simulink model "SLUGS2"  (R2015a)
settings: Solver=FixedStepDiscrete  StartTime=0.0  StopTime=10.0  FixedStep=T  RelTol=1e-3
PreLoadFcn:
  | %T = 0.0025;
  | MavlinkBus;
  | mcuInit;
  | % Baro Altitude Computation
  | % =========================
  | %basePressure = 98192.64;
  | %baseTemp = 288.215;
  | %lapseRate = -0.00198122;
  | %baseHeight = 0;
values from neighbouring files (symbols this model uses):
  apSampleTime = 0.01    [mcuInit.m]
  latlong_WP = 1    [mcuInit.m]
  mavlink_attitude_t = Simulink.Bus    [MavlinkBusMarcello.m]
  mavlink_gps_raw_int_t = Simulink.Bus    [MavlinkBus.m]    (also in MavlinkBusMarcello.m)
  mavlink_raw_imu_t = Simulink.Bus    [MavlinkBus.m]    (also in MavlinkBusMarcello.m)
  mavlink_scaled_pressure_t = Simulink.Bus    [MavlinkBus.m]    (also in MavlinkBusMarcello.m)
  mavlink_servo_output_raw_t = Simulink.Bus    [MavlinkBusMarcello.m]
  mavlink_slugs_navigation_t = Simulink.Bus    [MavlinkBusMarcello.m]
  mavlink_sys_status_t = Simulink.Bus    [MavlinkBus.m]    (also in MavlinkBusMarcello.m)
  SYS_ID_DEF = mpt.Parameter    [mcuInit.m]
  T = 0.01    [mcuInit.m]
  Xpoints = [0 0]    [mcuInit.m]
  Ypoints = [0 0]    [mcuInit.m]
  Zpoints = [0 0]    [mcuInit.m]
undefined symbols (not defined in the file or in its folder): A0, A14, A15, A2, A3, A4, A5, A6, accBiasRateLimit, B0, bankCommandLimit, barAdjust, baroCutoff, baroCutTemp, baseHeight, baseTemp, bdt, cubeAccelGain16405, cubeGyroGain16405, cubeMagGain16405, D0, D11, D7, D8, daLimit, data, daTrimMax, daTrimMin, deLimit, deTrimMax, deTrimMin, drLimit, drTrimMax, drTrimMin, dtLimit, dtTrimMax, dtTrimMin, F2, F3, G0, G13, G15, gaind, GS_location, gyroBiasRateLimit, imuOffset_xacc, imuOffset_xgyro, imuOffset_yacc, imuOffset_ygyro, imuOffset_zacc, imuOffset_zgyro, IPStar, ISA_g, Max, maxAcc, MaxDwnPthStar, maxDynPressure, maxEta, mdt, mlParamInterface ... (+34)
undefined symbols (not defined in the file): baroOffset, baroScale, barTGain1, barTGain2, barTMean1, barTMean2, bda, bde, bdr, bICda, bICde, bICdr, bICdt, derivativesConstant, lapseRate, lowRateSensorCutoff, mainSensorCutoff, mda, mde, mdr, mICda, mICde, mICdr, mICdt, pitotOffset, pitotScale, pitTGain1, pitTGain2, pitTMean1, pitTMean2, powerOffset, powerScale, pressureSensorCutoff, tempOffset, tempScale, vzCutoff, xCutoff, yCutoff
libraries: MCHP_Blockset x151, simulink x84, SLUGS_Library x31, aerolibconvert2 x6, aerolibutil x4, aerolibtransform2 x3, dspmtrx3 x2, aerolibobsolete x2
(part 16 of 24)

== system SLUGS2/Sensor_Data_Adapter/Sensor Suite/ GPS is Ublox ==
  Produce the GPS Main Data and update the AP State (lat lon hei cog sog) [gpsUblox.c]1 : MCHP_Blockset/User Functions/C Function Call  ParseFilesChkbx=on  ListFunctions1=Custom Function  Function1=void getGpsUbloxData(real32_T* y1);  AddHeaderDeclaration=on  Function1Type=when block is updated (default)  FctReturnBlockOut=off  Fct1BlockOut=y1[5]  DataCollected="s.chksm=reshape({ '638530-ספט-2016 08:52:24','251930-ספט-2016 08:52:57','1656312-אוק-2016 11:02:56','3862408-אוק-2016 23:39:15','360330-ספט-2016 08:52:57','7293730-ספט-2016 08:52:57','954930-ספט-2016 08:52:57','296108-אוק-2016 23:39:15','278130-ספט-2016 08:52:57','556030-ספט-2016 08:52:57','963230-ספט-2016 08:52:57','1122730-ספט-2016 08:52:57','372430-ספט-2016 08:52:57','998830-ספט-2016 08:52:57','522508-אוק-2016 23:39:15'},1,15);s.File1=reshape({ '  void  newCircBuffer(CBRef cB)','  void  freeCircBuffer(CBRef* cB)','  void  freeCircBuffer(CBRef* cB)',' unsigned int  getLength(CBRef cB)','  int  readHead(CBRef cB)','  int  readTail(CBRef cB)',' unsigned char  peak(CBRef cB)',' unsigned char  readFront(CBRef cB)',' unsigned char  writeBack(CBRef cB, unsigned char data)','  void  makeEmpty(CBRef cB)','  void  printCircBuf(CBRef cB)'},1,11);s.File2=reshape({ '  void  uartBufferInit(void)','  void  __attribute__((__interrupt__, no_auto_psv)) _U4RXInterrupt(void)','  void  getGPSRawData(unsigned char* gpsBuffer)',' unsigned char  isGPSNovatel(void)'},1,4);s.File3=reshape({ '  char  hex2char(char halfhex)','  float  degMinToDeg(unsigned char degrees, float minutes)',' unsigned char  gpsUbloxSeparate(unsigned char* outStream)','  void  gpsUbloxParse(void)','  void  getGpsUbloxMainData(float* data)','  void  getGpsUbloxData(float* data)','  char  gpSmbl(char symbl)',' unsigned char  myTokenizer(char* stringToTokenize, char token, char * returnToken)','  void  parseRMC(unsigned char* stream)','  void  parseGGA(unsigned char* stream)',' unsigned char  getChecksum(unsigned char* sentence, unsigned char size)','  void  gpsDebugMsg(unsigned char buf)'},1,12);s.File4=reshape({ '  void  uartMavlinkBufferInit(void)','  void __attribute__((__interrupt__,__auto_psv__)) _U1RXInterrupt(void)','  uint8_t  isFinite(float s)','  void  InitParameterInterface(void)','  void  protDecodeMavlink(void)','  uint16_t  MissionInterfaceResponse(uint8_t system_id, uint8_t component_id)','  uint16_t  ParameterInterfaceResponse(uint8_t system_id, uint8_t component_id)','  uint16_t  PackHeartBeat(uint8_t system_id, uint8_t component_id)','  uint16_t  PackTextMsg(uint8_t system_id, uint8_t component_id, unsigned char buf)','  uint16_t  PackRawIMU(uint8_t system_id, uint8_t component_id, mavlink_raw_imu_t mlRawIMUData ,uint32_t time_usec)','  uint16_t  PackRawAttitude(uint8_t system_id, uint8_t component_id, mavlink_attitude_t mlAttitudeData ,uint32_t time_usec)','  uint16_t  PackGpsRawInt(uint8_t system_id, uint8_t component_id, mavlink_gps_raw_int_t mlRawGpsDataInt ,uint32_t time_usec)','  uint16_t  PackScaledPressure(uint8_t system_id, uint8_t component_id, mavlink_scaled_pressure_t mlAirData ,uint32_t time_usec)','  uint16_t  PackSysStatus(uint8_t system_id, uint8_t component_id, mavlink_sys_status_t mlSysStatus)','  uint16_t  PackRawServo(uint8_t system_id, uint8_t component_id, mavlink_servo_output_raw_t mlPwmCommands ,uint32_t time_usec)','  uint16_t  HIL_PackRawServo(uint8_t system_id, uint8_t component_id, mavlink_servo_output_raw_t mlPwmCommands ,uint32_t time_usec)','  uint16_t  PackRawRC(uint8_t system_id, uint8_t component_id, mavlink_rc_channels_raw_t mlRC_Commands ,uint32_t time_usec)','  uint16_t  PackVFR_HUD(uint8_t system_id, uint8_t component_id, mavlink_vfr_hud_t mlVfr_hud ,uint32_t time_usec)','  char  sendQGCDebugMessage(const char * dbgMessage, char severity, unsigned char* bytesToAdd, char positionStart)','  void  TxN_Data_OverU1(uint16_t N)','  void  TxN_Data_OverU4(uint16_t N)'},1,21);s.File5=reshape({ '  float  myAtan2(float num, float denom)','  float  myPow(float x, float toTheN)','  float  mySqrt(float x)','  float  myAbs(float x)','  float  myAtan(float x)','  float  myAsin(float x)','  float  mySin(float x)','  float  myCos(float x)','  float  myTan(float x)','  float  myAcos(float x)','  float  myExp(float x)','  void  hugeDelay(void)','  void  smallDelay(void)','  void  tinyDelay(void)','  void  printToUart2(const char *fmt, ...)'},1,15);s.File6=reshape({ '  void  sendTelemetryMavlink(unsigned char* dataOut)','  void  uart2Init(void)','  void  gsRead(unsigned char* gsChunk)','  void  prepareTelemetryMavlink(unsigned char* dataOut)','  void  prepareTelemetryMavlink(unsigned char* dataOut)','  void  sendTelemetryMavlink(unsigned char* dataOut)','  void  copyBufferToDMA1(unsigned char size)','  void  send2GS(unsigned char* protData)','  uint8_t  clearWaypointsFrom(uint8_t startingWp)','  void  addMessageToSpiOut(mavlink_message_t* msg)'},1,10);s.File7={ '  void  populateParameterInterface(void)'};s.File8={ '  void  mavlinkInit(void)'};s.File9=reshape({ '  void  updatePWM(unsigned short * PWMData)','  void  updatePWMTrim(unsigned short PWMData, unsigned char channel)','  void  updateLoad(uint8_t mcuLoad)','  void  updateEuler(float* newEuler)','  void  updatePQR(float* newPQR)',' unsigned char  getHilOnOff(void)','  uint8_t  getLightsOnOff(void)','  uint8_t  getLightsDayNight(void)','  void  updateVISensor(uint16_t* data)','  void  updatePTZ(int16_t* ptz)'},1,10);s.File10=reshape({ '  void  updateRawADCData(int16_t* adcData)','  void  updateAirData(float* airData)','  void  updateLoadData(uint8_t load, uint16_t mvPower)','  void  updateAttitude(float * attitudeData)','  void  getGSLocation(float* altLatLon)','  void  updateTimeStamp(uint32_t timeSt)','  void  updatePosition(float * posData)','  void  updatePilotConsole(uint16_t * pilData)','  void  updateDiagnosticFl(float* diagFl)','  void  updateDiagnosticSh(int16_t* diagSh)','  void  updateBias(float * biasData)','  void  updateSensorData(float* sens)','  uint8_t  isFixValid(void)','  void  updateSensorDiag(float* diag)'},1,14);s.File11=reshape({ '  void  gpsInit(void)','  void  gpsParse(uint8_t* dataStream)','  void  updateStatus(uint8_t* completeMessage)','  void  updatePositionData(uint8_t* completeMessage)','  void  updateVelocityData(uint8_t* completeMessage)','  void  updateTimeData(uint8_t* completeMessage)','  void  getGpsMainData(float* data)','  uint32_t  CRC32Value(int32_t i)','  uint32_t  CalculateBlockCRC32(uint32_t ulCount, uint8_t *ucBuffer)','  uint16_t  charsToUint16(uint8_t* data)','  uint32_t  charsToUint32(uint8_t* data)','  float  charsToFloat(uint8_t* data)','  double  charsToDouble(uint8_t* data)'},1,13);s.File12=reshape({ '  void  getMidLevelCommands(float* commands)',' unsigned char  isApManual(uint16_t failsafe)','  float  getParamIdx(unsigned char idx)','  void  getRangeOfParams(uint8_t startIdx, uint8_t endIdx, float* parameters)','  float  getDynamic(void)','  void  getAttitude(float* attitude)','  void  getXYZ(float* xyz)','  void  getVned(float* xyz)','  uint8_t  getMaxWp(void)',' unsigned char  isWpFly(void)',' unsigned char  isPassthrough(void)','  void  setDiagnosticFloat(float * flValues)','  void  setDiagnosticShort(int16_t* shValues)','  void  getWP(unsigned char idx, float* WPpos)','  void  setLogFloat1(float * flValues)','  void  setLogFloat2(float * flValues)',' unsigned char  getApControlType(void)',' unsigned char  getPassValues(uint8_t* pasVals)','  void  setCurrentCommands(float airSpeed)','  void  getCurrentGPSPos(float* latLonAlt)','  void  setNavLong(float* values)','  void  setNavLat(float* values)','  void  setNavNav(float* values)','  void  getAccels(float * accels)','  void  getAccBias(float * bias)','  void  getRTB(uint8_t* rtb)','  void  getMobileLocation(float* loc)','  uint8_t  getNavMode(void)','  void  getISRLocation(float* loc)','  uint8_t  getISRCameraOption1(void)',' unsigned short  meanFilter5(unsigned short * values)','  uint8_t  justEnabled(uint8_t enableValue, uint8_t index)',' unsigned char  quickSort(unsigned short *arr, char elements)'},1,33);s.File13=reshape({ '  void  hilRead(unsigned char* hilChunk)','  void  hil_getRawRead(short * rawData)','  void  hil_getVned(float* vned)','  void  hil_getEuler(float* euler)','  void  hil_getRates(float* pqr)','  void  hil_getXYZ(float* xyz)',' unsigned int  hil_getTs(void)','  void  protDecodeHil(uint8_t* dataIn)'},1,8);s.File14=reshape({ '  void  cubeInit(void)','  void  getCubeData(short * cubeData)','  void  updateCubeData(void)','  int16_t  averageData(int16_t* theData, uint8_t count)',' unsigned short  write2Cube(unsigned short data2Send)','  short  convert14BitToShort(short wordData)','  short  convert12BitToShort(short wordData)',' unsigned char  isCube16405(void)'},1,8);s.File15=reshape({ '  void  uartMavlinkBufferInit(void)','  uint16_t  PackHeartBeat(uint8_t system_id, uint8_t component_id)','  uint16_t  PackRawServo(uint8_t system_id, uint8_t component_id, mavlink_servo_output_raw_t mlPwmCommands ,uint32_t time_usec)','  uint16_t  HIL_PackRawServo(uint8_t system_id, uint8_t component_id, mavlink_servo_output_raw_t mlPwmCommands ,uint32_t time_usec)','  uint16_t  PackRawRC(uint8_t system_id, uint8_t component_id, mavlink_rc_channels_raw_t mlRC_Commands, uint32_t time_usec)','  uint16_t  PackVFR_HUD(uint8_t system_id, uint8_t component_id, mavlink_vfr_hud_t mlVfr_hud, uint32_t time_usec)','  uint16_t  PackRawIMU(uint8_t system_id, uint8_t component_id, mavlink_raw_imu_t mlRawIMUData ,uint32_t time_usec)','  uint16_t  PackRawAttitude(uint8_t system_id, uint8_t component_id, mavlink_attitude_t mlAttitudeData ,uint32_t time_usec)','  char  sendQGCDebugMessage(const char * dbgMessage, char severity, unsigned char* bytesToAdd, char positionStart)','  uint16_t  PackGpsRawInt(uint8_t system_id, uint8_t component_id, mavlink_gps_raw_int_t mlRawGpsDataInt, uint32_t time_usec)','  uint16_t  PackScaledPressure(uint8_t system_id, uint8_t component_id, mavlink_scaled_pressure_t mlAirData, uint32_t time_usec)','  uint16_t  PackSysStatus(uint8_t system_id, uint8_t component_id, mavlink_sys_status_t mlSysStatus)'},1,12);"  ORDERING=None  SampleTime=.01  MCHP_MASTERLINK=|  PinDigitalInput=[]  PinDigitalOutput=[]  PinAnalogInput=[]
      | SLUGS2/Microchip Master
      | AUAV V3 Board
      | Busy Flag on D2 (RA6)
  GPS Main : Outport
  wires:
  Produce the GPS Main Data and update the AP State (lat lon hei cog sog) [gpsUblox.c]1/1 -> GPS Main/1

== system SLUGS2/Sensor_Data_Adapter/Sensor Suite/ADIS16405 Signal Cond  ==
  Gyro Raw : Inport
  Accel Raw : Inport  Port=2
  Mag Raw : Inport  Port=3
  "3D Tustin Lowpass, Auto Initial Condition" : Subsystem  mask(Tustin1stOrderLowpassAutoInitialCondition){f=mainSensorCutoff, T=T}
      mask prompts: f "Lowpass Frequency"; T "Sample Time"
      mask help: Takes a 3db rolloff frequency (in Hz, NOT radians/s) and a sample time. Performs a symbolic Tustin conversion and implements in a discrete filter. The initial output of the filter is set by the first sample.
      mask Help: Enter the desired 3db rolloff frequency in Hz and the sample time. Initial conditions are sampled automatically.
      mask Display: fprintf('%.2f Hz lowpass (3D)',f)
  "3D Tustin Lowpass, Auto Initial Condition1" : Subsystem  mask(Tustin1stOrderLowpassAutoInitialCondition){f=mainSensorCutoff, T=T}
      mask prompts: f "Lowpass Frequency"; T "Sample Time"
      mask help: Takes a 3db rolloff frequency (in Hz, NOT radians/s) and a sample time. Performs a symbolic Tustin conversion and implements in a discrete filter. The initial output of the filter is set by the first sample.
      mask Help: Enter the desired 3db rolloff frequency in Hz and the sample time. Initial conditions are sampled automatically.
      mask Display: fprintf('%.2f Hz lowpass (3D)',f)
  "3D Tustin Lowpass, Auto Initial Condition2" : Subsystem  mask(Tustin1stOrderLowpassAutoInitialCondition){f=mainSensorCutoff, T=T}
      mask prompts: f "Lowpass Frequency"; T "Sample Time"
      mask help: Takes a 3db rolloff frequency (in Hz, NOT radians/s) and a sample time. Performs a symbolic Tustin conversion and implements in a discrete filter. The initial output of the filter is set by the first sample.
      mask Help: Enter the desired 3db rolloff frequency in Hz and the sample time. Initial conditions are sampled automatically.
      mask Display: fprintf('%.2f Hz lowpass (3D)',f)
  Data Type Conversion1 : DataTypeConversion  OutDataTypeStr=double
  Data Type Conversion2 : DataTypeConversion  OutDataTypeStr=double
  Data Type Conversion3 : DataTypeConversion  OutDataTypeStr=single
  Data Type Conversion5 : DataTypeConversion  OutDataTypeStr=double
  Data Type Conversion6 : DataTypeConversion  OutDataTypeStr=single
  Data Type Conversion7 : DataTypeConversion  OutDataTypeStr=single
  Divide : Product  OutDataTypeStr=single
  Divide1 : Product  OutDataTypeStr=single
  Divide2 : Product  OutDataTypeStr=single
  Gyro Gains : Constant  Value=cubeGyroGain16405  OutDataTypeStr=single
  Gyro Gains1 : Constant  Value=cubeAccelGain16405  OutDataTypeStr=single
  Gyro Gains2 : Constant  Value=cubeMagGain16405  OutDataTypeStr=single
  Rotate Cube Axis : Subsystem
  "Rotate Cube Axis " : Subsystem
  "Rotate Cube Axis  " : Subsystem
  Omega (rad/s) : Outport
  Accel (m/s^2) : Outport  Port=2
  Mags (mG) : Outport  Port=3
  wires:
  Gyro Gains/1 -> Divide/2
  Divide/1 -> Rotate Cube Axis/1(Raw)
  Divide1/1 -> "Rotate Cube Axis "/1(Raw)
  "Rotate Cube Axis "/1(Rotated) -> Data Type Conversion1/1
  Gyro Gains1/1 -> Divide1/2
  Gyro Raw/1 -> Divide/1
  Data Type Conversion2/1 -> "3D Tustin Lowpass, Auto Initial Condition"/1(In1)
  "3D Tustin Lowpass, Auto Initial Condition"/1(Out1) -> Data Type Conversion7/1
  Data Type Conversion7/1 -> Omega (rad/s)/1
  Rotate Cube Axis/1(Rotated) -> Data Type Conversion2/1
  Data Type Conversion1/1 -> "3D Tustin Lowpass, Auto Initial Condition1"/1(In1)
  "3D Tustin Lowpass, Auto Initial Condition1"/1(Out1) -> Data Type Conversion3/1
  Data Type Conversion3/1 -> Accel (m/s^2)/1
  Accel Raw/1 -> Divide1/1
  Divide2/1 -> "Rotate Cube Axis  "/1(Raw)
  Data Type Conversion5/1 -> "3D Tustin Lowpass, Auto Initial Condition2"/1(In1)
  "3D Tustin Lowpass, Auto Initial Condition2"/1(Out1) -> Data Type Conversion6/1
  Data Type Conversion6/1 -> Mags (mG)/1
  "Rotate Cube Axis  "/1(Rotated) -> Data Type Conversion5/1
  Mag Raw/1 -> Divide2/1
  Gyro Gains2/1 -> Divide2/2

== system SLUGS2/Sensor_Data_Adapter/Sensor Suite/Compute CPU Load ==
  Calculus Time Step1 : MCHP_Blockset/Profiling/MCU Load  MCULoadPin=Dynamic Options  MCULoadPin_TXT=None  MCULoadMeasure=on  TIMER_Resolution=Dynamic Options  TIMER_Resolution_TXT="Resol: 0.9143(us)  -  Max: 59.9(ms)"  MCHP_TIMER_REQUEST={MCU_Load}{MCU_Load}21:5:0:0:[]:4194304;  MCHP_TIMER_RESULT=[3 65535 ]  MCHP_MASTERLINK=|  MCHP_COMPILED_INFO="CompiledSampleTime= [0.01   0 ];CompiledInportDataTypes=[ ];CompiledInportDataWidth=[];"  Info="Timer 3:  Resol: 914.2857143(ns)  -  Max: 59.9186(ms)"  SampleTime=.01
      | SLUGS2/Microchip Master
      | AUAV V3 Board
      | Busy Flag on D2 (RA6)
  Calculus Time Step2 : MCHP_Blockset/Profiling/MCU Overload  MCUOverloadBlockOutput=on  MCUOverLoadPin=Dynamic Options  MCUOverLoadPin_TXT=None  MCHP_MASTERLINK=|  SampleTime=.01
      | SLUGS2/Microchip Master
      | AUAV V3 Board
      | Busy Flag on D2 (RA6)
  Data Type Conversion1 : DataTypeConversion  OutDataTypeStr=single
  Data Type Conversion12 : DataTypeConversion  OutDataTypeStr=uint8
  Data Type Conversion2 : DataTypeConversion  OutDataTypeStr=single
  Divide : Product  Inputs=*/  OutDataTypeStr=double
  Gain : Gain  Gain=100
  Rounding Function : Rounding
  Load (%) : Outport
  wires:
  Calculus Time Step1/1 -> Data Type Conversion2/1
  Calculus Time Step2/1 -> Data Type Conversion1/1
  Divide/1 -> Gain/1
  Rounding Function/1 -> Data Type Conversion12/1
  Data Type Conversion1/1 -> Divide/2
  Data Type Conversion2/1 -> Divide/1
  Data Type Conversion12/1 -> Load (%)/1
  Gain/1 -> Rounding Function/1

== system SLUGS2/Sensor_Data_Adapter/Sensor Suite/If no HIL then Read all the Sensors ==
  Enable : EnablePort
  Bus Creator : BusCreator  Commented=on  Inputs=3
  Bus Creator1 : BusCreator  Commented=on  Inputs=3
  Bus Creator2 : BusCreator  Commented=on  Inputs=3
  Bus Creator3 : BusCreator  Commented=on  DialogController=Simulink.DDGSource_BusCreator  Inputs=5
  Constant : Constant  Commented=on  Value=[1 1 1 1 1]
  Constant1 : Constant  Value=[1 1 1 1 1]
  Constant2 : Constant  Value=[1 1 1 1 1]
  Constant3 : Constant  Commented=on  Value=[1 1 1 1 1]
  Data Type Conversion{,1..3} (4 alike) : DataTypeConversion  OutDataTypeStr=int16
  Data Type Conversion{4..6,8..9} (5 alike) : DataTypeConversion  Commented=on  OutDataTypeStr=single
  Demux : Demux  Outputs=6
  Demux1 : Demux  Outputs=3
  Demux2 : Demux  Outputs=[6 3 1]
  Embedded MATLAB Function : MATLAB Function  Commented=on  TreatAsAtomicUnit=on
  Embedded MATLAB Function1 : MATLAB Function  TreatAsAtomicUnit=on
  Embedded MATLAB Function2 : MATLAB Function  TreatAsAtomicUnit=on
  Embedded MATLAB Function3 : MATLAB Function  Commented=on  TreatAsAtomicUnit=on
  From1 : From  Commented=on  GotoTag=isNovatel
  From4 : From  Commented=on  GotoTag=isNovatel
  Get Raw IMU : DataStoreRead  Commented=on  DialogController=Simulink.DDGSource  DataStoreName=mlRawImuData  DataStoreElements=mlRawIMU.xgyro#mlRawIMU.ygyro#mlRawIMU.zgyro#mlRawIMU.xacc#mlRawIMU.yacc#mlRawIMU.zacc#mlRawIMU.xmag#mlRawIMU.ymag#mlRawIMU.zmag
  Get RawGpsInt : DataStoreRead  Commented=on  DialogController=Simulink.DDGSource  DataStoreName=mlGpsData  DataStoreElements=mlGpsData.lat#mlGpsData.lon#mlGpsData.alt#mlGpsData.cog#mlGpsData.vel
  Get mlAirData1 : DataStoreRead  DialogController=Simulink.DDGSource  DataStoreName=mlAirData  DataStoreElements=mlAirData.press_abs
  Get mlAirData2 : DataStoreRead  DialogController=Simulink.DDGSource  DataStoreName=mlAirData  DataStoreElements=mlAirData.temperature
  Goto1 : Goto  Commented=on  GotoTag=isNovatel
  Is the GPS Novatel or Ublox? [gpsPort.c]1 : MCHP_Blockset/User Functions/C Function Call  ParseFilesChkbx=on  ListFunctions1=Custom Function  Function1=uint8_T isGPSNovatel();  AddHeaderDeclaration=on  Function1Type=when block is updated (default)  FctReturnBlockOut=on  DataCollected="s.chksm=reshape({ '638529-אוק-2016 01:00:36','251929-אוק-2016 01:00:36','1689429-אוק-2016 01:00:36','4250714-אוק-2016 08:45:05','360329-אוק-2016 01:00:36','7293729-אוק-2016 01:00:36','954929-אוק-2016 01:00:36','296129-אוק-2016 01:00:36','278129-אוק-2016 01:00:36','556029-אוק-2016 01:00:36','963229-אוק-2016 01:00:36','1122729-אוק-2016 01:00:36','372429-אוק-2016 01:00:36','998829-אוק-2016 01:00:36','536514-אוק-2016 08:45:05'},1,15);s.File1=reshape({ '  void  newCircBuffer(CBRef cB)','  void  freeCircBuffer(CBRef* cB)','  void  freeCircBuffer(CBRef* cB)',' unsigned int  getLength(CBRef cB)','  int  readHead(CBRef cB)','  int  readTail(CBRef cB)',' unsigned char  peak(CBRef cB)',' unsigned char  readFront(CBRef cB)',' unsigned char  writeBack(CBRef cB, unsigned char data)','  void  makeEmpty(CBRef cB)','  void  printCircBuf(CBRef cB)'},1,11);s.File2=reshape({ '  void  uartBufferInit(void)','  void  __attribute__((__interrupt__, no_auto_psv)) _U4RXInterrupt(void)','  void  getGPSRawData(unsigned char* gpsBuffer)',' unsigned char  isGPSNovatel(void)'},1,4);s.File3=reshape({ '  char  hex2char(char halfhex)','  float  degMinToDeg(unsigned char degrees, float minutes)',' unsigned char  gpsUbloxSeparate(unsigned char* outStream)','  void  gpsUbloxParse(void)','  void  getGpsUbloxMainData(float* data)','  void  getGpsUbloxData(float* data)','  char  gpSmbl(char symbl)',' unsigned char  myTokenizer(char* stringToTokenize, char token, char * returnToken)','  void  parseRMC(unsigned char* stream)','  void  parseGGA(unsigned char* stream)',' unsigned char  getChecksum(unsigned char* sentence, unsigned char size)','  void  gpsDebugMsg(unsigned char buf)'},1,12);s.File4=reshape({ '  void  uartMavlinkBufferInit(void)','  void __attribute__((__interrupt__,__auto_psv__)) _U1RXInterrupt(void)','  uint8_t  isFinite(float s)','  void  InitParameterInterface(void)','  void  protDecodeMavlink(void)','  uint16_t  MissionInterfaceResponse(uint8_t system_id, uint8_t component_id)','  uint16_t  ParameterInterfaceResponse(uint8_t system_id, uint8_t component_id)','  uint16_t  PackHeartBeat(uint8_t system_id, uint8_t component_id)','  uint16_t  PackTextMsg(uint8_t system_id, uint8_t component_id, unsigned char buf)','  uint16_t  PackRawIMU(uint8_t system_id, uint8_t component_id, mavlink_raw_imu_t mlRawIMUData ,uint32_t time_usec)','  uint16_t  PackRawAttitude(uint8_t system_id, uint8_t component_id, mavlink_attitude_t mlAttitudeData ,uint32_t time_usec)','  uint16_t  PackPosXYZ_Sol(uint8_t system_id, uint8_t component_id, mavlink_local_position_ned_t mlLocalPositionSol ,uint32_t time_usec)','  uint16_t  PackGpsRawInt(uint8_t system_id, uint8_t component_id, mavlink_gps_raw_int_t mlRawGpsDataInt ,uint32_t time_usec)','  uint16_t  PackScaledPressure(uint8_t system_id, uint8_t component_id, mavlink_scaled_pressure_t mlAirData ,uint32_t time_usec)','  uint16_t  PackSysStatus(uint8_t system_id, uint8_t component_id, mavlink_sys_status_t mlSysStatus)','  uint16_t  PackRawServo(uint8_t system_id, uint8_t component_id, mavlink_servo_output_raw_t mlPwmCommands ,uint32_t time_usec)','  uint16_t  HIL_PackRawServo(uint8_t system_id, uint8_t component_id, mavlink_servo_output_raw_t mlPwmCommands ,uint32_t time_usec)','  uint16_t  PackRawRC(uint8_t system_id, uint8_t component_id, mavlink_rc_channels_raw_t mlRC_Commands ,uint32_t time_usec)','  uint16_t  PackVFR_HUD(uint8_t system_id, uint8_t component_id, mavlink_vfr_hud_t mlVfr_hud ,uint32_t time_usec)','  char  sendQGCDebugMessage(const char * dbgMessage, char severity, unsigned char* bytesToAdd, char positionStart)','  void  TxN_Data_OverU1(uint16_t N)','  void  TxN_Data_OverU4(uint16_t N)'},1,22);s.File5=reshape({ '  float  myAtan2(float num, float denom)','  float  myPow(float x, float toTheN)','  float  mySqrt(float x)','  float  myAbs(float x)','  float  myAtan(float x)','  float  myAsin(float x)','  float  mySin(float x)','  float  myCos(float x)','  float  myTan(float x)','  float  myAcos(float x)','  float  myExp(float x)','  void  hugeDelay(void)','  void  smallDelay(void)','  void  tinyDelay(void)','  void  printToUart2(const char *fmt, ...)'},1,15);s.File6=reshape({ '  void  sendTelemetryMavlink(unsigned char* dataOut)','  void  uart2Init(void)','  void  gsRead(unsigned char* gsChunk)','  void  prepareTelemetryMavlink(unsigned char* dataOut)','  void  prepareTelemetryMavlink(unsigned char* dataOut)','  void  sendTelemetryMavlink(unsigned char* dataOut)','  void  copyBufferToDMA1(unsigned char size)','  void  send2GS(unsigned char* protData)','  uint8_t  clearWaypointsFrom(uint8_t startingWp)','  void  addMessageToSpiOut(mavlink_message_t* msg)'},1,10);s.File7={ '  void  populateParameterInterface(void)'};s.File8={ '  void  mavlinkInit(void)'};s.File9=reshape({ '  void  updatePWM(unsigned short * PWMData)','  void  updatePWMTrim(unsigned short PWMData, unsigned char channel)','  void  updateLoad(uint8_t mcuLoad)','  void  updateEuler(float* newEuler)','  void  updatePQR(float* newPQR)',' unsigned char  getHilOnOff(void)','  uint8_t  getLightsOnOff(void)','  uint8_t  getLightsDayNight(void)','  void  updateVISensor(uint16_t* data)','  void  updatePTZ(int16_t* ptz)'},1,10);s.File10=reshape({ '  void  updateRawADCData(int16_t* adcData)','  void  updateAirData(float* airData)','  void  updateLoadData(uint8_t load, uint16_t mvPower)','  void  updateAttitude(float * attitudeData)','  void  getGSLocation(float* altLatLon)','  void  updateTimeStamp(uint32_t timeSt)','  void  updatePosition(float * posData)','  void  updatePilotConsole(uint16_t * pilData)','  void  updateDiagnosticFl(float* diagFl)','  void  updateDiagnosticSh(int16_t* diagSh)','  void  updateBias(float * biasData)','  void  updateSensorData(float* sens)','  uint8_t  isFixValid(void)','  void  updateSensorDiag(float* diag)'},1,14);s.File11=reshape({ '  void  gpsInit(void)','  void  gpsParse(uint8_t* dataStream)','  void  updateStatus(uint8_t* completeMessage)','  void  updatePositionData(uint8_t* completeMessage)','  void  updateVelocityData(uint8_t* completeMessage)','  void  updateTimeData(uint8_t* completeMessage)','  void  getGpsMainData(float* data)','  uint32_t  CRC32Value(int32_t i)','  uint32_t  CalculateBlockCRC32(uint32_t ulCount, uint8_t *ucBuffer)','  uint16_t  charsToUint16(uint8_t* data)','  uint32_t  charsToUint32(uint8_t* data)','  float  charsToFloat(uint8_t* data)','  double  charsToDouble(uint8_t* data)'},1,13);s.File12=reshape({ '  void  getMidLevelCommands(float* commands)',' unsigned char  isApManual(uint16_t failsafe)','  float  getParamIdx(unsigned char idx)','  void  getRangeOfParams(uint8_t startIdx, uint8_t endIdx, float* parameters)','  float  getDynamic(void)','  void  getAttitude(float* attitude)','  void  getXYZ(float* xyz)','  void  getVned(float* xyz)','  uint8_t  getMaxWp(void)',' unsigned char  isWpFly(void)',' unsigned char  isPassthrough(void)','  void  setDiagnosticFloat(float * flValues)','  void  setDiagnosticShort(int16_t* shValues)','  void  getWP(unsigned char idx, float* WPpos)','  void  setLogFloat1(float * flValues)','  void  setLogFloat2(float * flValues)',' unsigned char  getApControlType(void)',' unsigned char  getPassValues(uint8_t* pasVals)','  void  setCurrentCommands(float airSpeed)','  void  getCurrentGPSPos(float* latLonAlt)','  void  setNavLong(float* values)','  void  setNavLat(float* values)','  void  setNavNav(float* values)','  void  getAccels(float * accels)','  void  getAccBias(float * bias)','  void  getRTB(uint8_t* rtb)','  void  getMobileLocation(float* loc)','  uint8_t  getNavMode(void)','  void  getISRLocation(float* loc)','  uint8_t  getISRCameraOption1(void)',' unsigned short  meanFilter5(unsigned short * values)','  uint8_t  justEnabled(uint8_t enableValue, uint8_t index)',' unsigned char  quickSort(unsigned short *arr, char elements)'},1,33);s.File13=reshape({ '  void  hilRead(unsigned char* hilChunk)','  void  hil_getRawRead(short * rawData)','  void  hil_getVned(float* vned)','  void  hil_getEuler(float* euler)','  void  hil_getRates(float* pqr)','  void  hil_getXYZ(float* xyz)',' unsigned int  hil_getTs(void)','  void  protDecodeHil(uint8_t* dataIn)'},1,8);s.File14=reshape({ '  void  cubeInit(void)','  void  getCubeData(short * cubeData)','  void  updateCubeData(void)','  int16_t  averageData(int16_t* theData, uint8_t count)',' unsigned short  write2Cube(unsigned short data2Send)','  short  convert14BitToShort(short wordData)','  short  convert12BitToShort(short wordData)',' unsigned char  isCube16405(void)'},1,8);s.File15=reshape({ '  void  uartMavlinkBufferInit(void)','  uint16_t  PackHeartBeat(uint8_t system_id, uint8_t component_id)','  uint16_t  PackRawServo(uint8_t system_id, uint8_t component_id, mavlink_servo_output_raw_t mlPwmCommands ,uint32_t time_usec)','  uint16_t  HIL_PackRawServo(uint8_t system_id, uint8_t component_id, mavlink_servo_output_raw_t mlPwmCommands ,uint32_t time_usec)','  uint16_t  PackRawRC(uint8_t system_id, uint8_t component_id, mavlink_rc_channels_raw_t mlRC_Commands, uint32_t time_usec)','  uint16_t  PackVFR_HUD(uint8_t system_id, uint8_t component_id, mavlink_vfr_hud_t mlVfr_hud, uint32_t time_usec)','  uint16_t  PackRawIMU(uint8_t system_id, uint8_t component_id, mavlink_raw_imu_t mlRawIMUData ,uint32_t time_usec)','  uint16_t  PackRawAttitude(uint8_t system_id, uint8_t component_id, mavlink_attitude_t mlAttitudeData ,uint32_t time_usec)','  uint16_t  PackPosXYZ_Sol(uint8_t system_id, uint8_t component_id, mavlink_local_position_ned_t mlLocalPositionSol ,uint32_t time_usec)','  char  sendQGCDebugMessage(const char * dbgMessage, char severity, unsigned char* bytesToAdd, char positionStart)','  uint16_t  PackGpsRawInt(uint8_t system_id, uint8_t component_id, mavlink_gps_raw_int_t mlRawGpsDataInt, uint32_t time_usec)','  uint16_t  PackScaledPressure(uint8_t system_id, uint8_t component_id, mavlink_scaled_pressure_t mlAirData, uint32_t time_usec)','  uint16_t  PackSysStatus(uint8_t system_id, uint8_t component_id, mavlink_sys_status_t mlSysStatus)'},1,13);"  ORDERING=None  SampleTime=.01  MCHP_MASTERLINK=|  PinDigitalInput=[]  PinDigitalOutput=[]  PinAnalogInput=[]
      | SLUGS2/Microchip Master
      | AUAV V3 Board
      | Busy Flag on D2 (RA6)
  Logical Operator : Logic  Operator=NOT  AllPortsSameDT=off  OutDataTypeStr=boolean
  Read the Cube Data [adisCube16405.c]1 : MCHP_Blockset/User Functions/C Function Call  ParseFilesChkbx=off  ListFunctions1=Custom Function  Function1=extern void getCubeData(int16_T* y1);  AddHeaderDeclaration=on  Function1Type=when block is updated (default)  FctReturnBlockOut=off  Fct1BlockOut=y1[10]  DataCollected=0  ORDERING=None  SampleTime=.01  MCHP_MASTERLINK=|  PinDigitalInput=[]  PinDigitalOutput=[]  PinAnalogInput=[]
      | SLUGS2/Microchip Master
      | AUAV V3 Board
      | Busy Flag on D2 (RA6)
  Switch2 : Switch  Commented=on  Criteria=u2 > Threshold  Threshold=0.3  ZeroCross=off
  Terminator : Terminator
  Update State AP ADC Data [updateSensorMcuState.c]1 : MCHP_Blockset/User Functions/C Function Call  ParseFilesChkbx=on  ListFunctions1=Custom Function  Function1=void updateRawADCData(int16_T* u1);  AddHeaderDeclaration=on  Function1Type=when block is updated (default)  Fct1BlockIn=u1  FctReturnBlockOut=on  DataCollected="s.chksm=reshape({ '638529-אוק-2016 01:00:36','251929-אוק-2016 01:00:36','1689429-אוק-2016 01:00:36','4250714-אוק-2016 08:45:05','360329-אוק-2016 01:00:36','7293729-אוק-2016 01:00:36','954929-אוק-2016 01:00:36','296129-אוק-2016 01:00:36','278129-אוק-2016 01:00:36','556029-אוק-2016 01:00:36','963229-אוק-2016 01:00:36','1122729-אוק-2016 01:00:36','372429-אוק-2016 01:00:36','998829-אוק-2016 01:00:36','536514-אוק-2016 08:45:05'},1,15);s.File1=reshape({ '  void  newCircBuffer(CBRef cB)','  void  freeCircBuffer(CBRef* cB)','  void  freeCircBuffer(CBRef* cB)',' unsigned int  getLength(CBRef cB)','  int  readHead(CBRef cB)','  int  readTail(CBRef cB)',' unsigned char  peak(CBRef cB)',' unsigned char  readFront(CBRef cB)',' unsigned char  writeBack(CBRef cB, unsigned char data)','  void  makeEmpty(CBRef cB)','  void  printCircBuf(CBRef cB)'},1,11);s.File2=reshape({ '  void  uartBufferInit(void)','  void  __attribute__((__interrupt__, no_auto_psv)) _U4RXInterrupt(void)','  void  getGPSRawData(unsigned char* gpsBuffer)',' unsigned char  isGPSNovatel(void)'},1,4);s.File3=reshape({ '  char  hex2char(char halfhex)','  float  degMinToDeg(unsigned char degrees, float minutes)',' unsigned char  gpsUbloxSeparate(unsigned char* outStream)','  void  gpsUbloxParse(void)','  void  getGpsUbloxMainData(float* data)','  void  getGpsUbloxData(float* data)','  char  gpSmbl(char symbl)',' unsigned char  myTokenizer(char* stringToTokenize, char token, char * returnToken)','  void  parseRMC(unsigned char* stream)','  void  parseGGA(unsigned char* stream)',' unsigned char  getChecksum(unsigned char* sentence, unsigned char size)','  void  gpsDebugMsg(unsigned char buf)'},1,12);s.File4=reshape({ '  void  uartMavlinkBufferInit(void)','  void __attribute__((__interrupt__,__auto_psv__)) _U1RXInterrupt(void)','  uint8_t  isFinite(float s)','  void  InitParameterInterface(void)','  void  protDecodeMavlink(void)','  uint16_t  MissionInterfaceResponse(uint8_t system_id, uint8_t component_id)','  uint16_t  ParameterInterfaceResponse(uint8_t system_id, uint8_t component_id)','  uint16_t  PackHeartBeat(uint8_t system_id, uint8_t component_id)','  uint16_t  PackTextMsg(uint8_t system_id, uint8_t component_id, unsigned char buf)','  uint16_t  PackRawIMU(uint8_t system_id, uint8_t component_id, mavlink_raw_imu_t mlRawIMUData ,uint32_t time_usec)','  uint16_t  PackRawAttitude(uint8_t system_id, uint8_t component_id, mavlink_attitude_t mlAttitudeData ,uint32_t time_usec)','  uint16_t  PackPosXYZ_Sol(uint8_t system_id, uint8_t component_id, mavlink_local_position_ned_t mlLocalPositionSol ,uint32_t time_usec)','  uint16_t  PackGpsRawInt(uint8_t system_id, uint8_t component_id, mavlink_gps_raw_int_t mlRawGpsDataInt ,uint32_t time_usec)','  uint16_t  PackScaledPressure(uint8_t system_id, uint8_t component_id, mavlink_scaled_pressure_t mlAirData ,uint32_t time_usec)','  uint16_t  PackSysStatus(uint8_t system_id, uint8_t component_id, mavlink_sys_status_t mlSysStatus)','  uint16_t  PackRawServo(uint8_t system_id, uint8_t component_id, mavlink_servo_output_raw_t mlPwmCommands ,uint32_t time_usec)','  uint16_t  HIL_PackRawServo(uint8_t system_id, uint8_t component_id, mavlink_servo_output_raw_t mlPwmCommands ,uint32_t time_usec)','  uint16_t  PackRawRC(uint8_t system_id, uint8_t component_id, mavlink_rc_channels_raw_t mlRC_Commands ,uint32_t time_usec)','  uint16_t  PackVFR_HUD(uint8_t system_id, uint8_t component_id, mavlink_vfr_hud_t mlVfr_hud ,uint32_t time_usec)','  char  sendQGCDebugMessage(const char * dbgMessage, char severity, unsigned char* bytesToAdd, char positionStart)','  void  TxN_Data_OverU1(uint16_t N)','  void  TxN_Data_OverU4(uint16_t N)'},1,22);s.File5=reshape({ '  float  myAtan2(float num, float denom)','  float  myPow(float x, float toTheN)','  float  mySqrt(float x)','  float  myAbs(float x)','  float  myAtan(float x)','  float  myAsin(float x)','  float  mySin(float x)','  float  myCos(float x)','  float  myTan(float x)','  float  myAcos(float x)','  float  myExp(float x)','  void  hugeDelay(void)','  void  smallDelay(void)','  void  tinyDelay(void)','  void  printToUart2(const char *fmt, ...)'},1,15);s.File6=reshape({ '  void  sendTelemetryMavlink(unsigned char* dataOut)','  void  uart2Init(void)','  void  gsRead(unsigned char* gsChunk)','  void  prepareTelemetryMavlink(unsigned char* dataOut)','  void  prepareTelemetryMavlink(unsigned char* dataOut)','  void  sendTelemetryMavlink(unsigned char* dataOut)','  void  copyBufferToDMA1(unsigned char size)','  void  send2GS(unsigned char* protData)','  uint8_t  clearWaypointsFrom(uint8_t startingWp)','  void  addMessageToSpiOut(mavlink_message_t* msg)'},1,10);s.File7={ '  void  populateParameterInterface(void)'};s.File8={ '  void  mavlinkInit(void)'};s.File9=reshape({ '  void  updatePWM(unsigned short * PWMData)','  void  updatePWMTrim(unsigned short PWMData, unsigned char channel)','  void  updateLoad(uint8_t mcuLoad)','  void  updateEuler(float* newEuler)','  void  updatePQR(float* newPQR)',' unsigned char  getHilOnOff(void)','  uint8_t  getLightsOnOff(void)','  uint8_t  getLightsDayNight(void)','  void  updateVISensor(uint16_t* data)','  void  updatePTZ(int16_t* ptz)'},1,10);s.File10=reshape({ '  void  updateRawADCData(int16_t* adcData)','  void  updateAirData(float* airData)','  void  updateLoadData(uint8_t load, uint16_t mvPower)','  void  updateAttitude(float * attitudeData)','  void  getGSLocation(float* altLatLon)','  void  updateTimeStamp(uint32_t timeSt)','  void  updatePosition(float * posData)','  void  updatePilotConsole(uint16_t * pilData)','  void  updateDiagnosticFl(float* diagFl)','  void  updateDiagnosticSh(int16_t* diagSh)','  void  updateBias(float * biasData)','  void  updateSensorData(float* sens)','  uint8_t  isFixValid(void)','  void  updateSensorDiag(float* diag)'},1,14);s.File11=reshape({ '  void  gpsInit(void)','  void  gpsParse(uint8_t* dataStream)','  void  updateStatus(uint8_t* completeMessage)','  void  updatePositionData(uint8_t* completeMessage)','  void  updateVelocityData(uint8_t* completeMessage)','  void  updateTimeData(uint8_t* completeMessage)','  void  getGpsMainData(float* data)','  uint32_t  CRC32Value(int32_t i)','  uint32_t  CalculateBlockCRC32(uint32_t ulCount, uint8_t *ucBuffer)','  uint16_t  charsToUint16(uint8_t* data)','  uint32_t  charsToUint32(uint8_t* data)','  float  charsToFloat(uint8_t* data)','  double  charsToDouble(uint8_t* data)'},1,13);s.File12=reshape({ '  void  getMidLevelCommands(float* commands)',' unsigned char  isApManual(uint16_t failsafe)','  float  getParamIdx(unsigned char idx)','  void  getRangeOfParams(uint8_t startIdx, uint8_t endIdx, float* parameters)','  float  getDynamic(void)','  void  getAttitude(float* attitude)','  void  getXYZ(float* xyz)','  void  getVned(float* xyz)','  uint8_t  getMaxWp(void)',' unsigned char  isWpFly(void)',' unsigned char  isPassthrough(void)','  void  setDiagnosticFloat(float * flValues)','  void  setDiagnosticShort(int16_t* shValues)','  void  getWP(unsigned char idx, float* WPpos)','  void  setLogFloat1(float * flValues)','  void  setLogFloat2(float * flValues)',' unsigned char  getApControlType(void)',' unsigned char  getPassValues(uint8_t* pasVals)','  void  setCurrentCommands(float airSpeed)','  void  getCurrentGPSPos(float* latLonAlt)','  void  setNavLong(float* values)','  void  setNavLat(float* values)','  void  setNavNav(float* values)','  void  getAccels(float * accels)','  void  getAccBias(float * bias)','  void  getRTB(uint8_t* rtb)','  void  getMobileLocation(float* loc)','  uint8_t  getNavMode(void)','  void  getISRLocation(float* loc)','  uint8_t  getISRCameraOption1(void)',' unsigned short  meanFilter5(unsigned short * values)','  uint8_t  justEnabled(uint8_t enableValue, uint8_t index)',' unsigned char  quickSort(unsigned short *arr, char elements)'},1,33);s.File13=reshape({ '  void  hilRead(unsigned char* hilChunk)','  void  hil_getRawRead(short * rawData)','  void  hil_getVned(float* vned)','  void  hil_getEuler(float* euler)','  void  hil_getRates(float* pqr)','  void  hil_getXYZ(float* xyz)',' unsigned int  hil_getTs(void)','  void  protDecodeHil(uint8_t* dataIn)'},1,8);s.File14=reshape({ '  void  cubeInit(void)','  void  getCubeData(short * cubeData)','  void  updateCubeData(void)','  int16_t  averageData(int16_t* theData, uint8_t count)',' unsigned short  write2Cube(unsigned short data2Send)','  short  convert14BitToShort(short wordData)','  short  convert12BitToShort(short wordData)',' unsigned char  isCube16405(void)'},1,8);s.File15=reshape({ '  void  uartMavlinkBufferInit(void)','  uint16_t  PackHeartBeat(uint8_t system_id, uint8_t component_id)','  uint16_t  PackRawServo(uint8_t system_id, uint8_t component_id, mavlink_servo_output_raw_t mlPwmCommands ,uint32_t time_usec)','  uint16_t  HIL_PackRawServo(uint8_t system_id, uint8_t component_id, mavlink_servo_output_raw_t mlPwmCommands ,uint32_t time_usec)','  uint16_t  PackRawRC(uint8_t system_id, uint8_t component_id, mavlink_rc_channels_raw_t mlRC_Commands, uint32_t time_usec)','  uint16_t  PackVFR_HUD(uint8_t system_id, uint8_t component_id, mavlink_vfr_hud_t mlVfr_hud, uint32_t time_usec)','  uint16_t  PackRawIMU(uint8_t system_id, uint8_t component_id, mavlink_raw_imu_t mlRawIMUData ,uint32_t time_usec)','  uint16_t  PackRawAttitude(uint8_t system_id, uint8_t component_id, mavlink_attitude_t mlAttitudeData ,uint32_t time_usec)','  uint16_t  PackPosXYZ_Sol(uint8_t system_id, uint8_t component_id, mavlink_local_position_ned_t mlLocalPositionSol ,uint32_t time_usec)','  char  sendQGCDebugMessage(const char * dbgMessage, char severity, unsigned char* bytesToAdd, char positionStart)','  uint16_t  PackGpsRawInt(uint8_t system_id, uint8_t component_id, mavlink_gps_raw_int_t mlRawGpsDataInt, uint32_t time_usec)','  uint16_t  PackScaledPressure(uint8_t system_id, uint8_t component_id, mavlink_scaled_pressure_t mlAirData, uint32_t time_usec)','  uint16_t  PackSysStatus(uint8_t system_id, uint8_t component_id, mavlink_sys_status_t mlSysStatus)'},1,13);"  ORDERING=None  SampleTime=.01  MCHP_MASTERLINK=|  PinDigitalInput=[]  PinDigitalOutput=[]  PinAnalogInput=[]
      | SLUGS2/Microchip Master
      | AUAV V3 Board
      | Busy Flag on D2 (RA6)
  if GPS is Novatel : Subsystem  Commented=on
  if GPS is Ublox : Subsystem
  myMux Fun : MATLAB Function  TreatAsAtomicUnit=on
  myMux Fun4 : MATLAB Function  TreatAsAtomicUnit=on
  Sensors : Outport
  GPS : Outport  Port=2
  wires:
  myMux Fun4/1(y) -> Sensors/1
  Demux2/1 -> Demux/1
  Demux/1 -> myMux Fun4/1(u1)
  Demux/2 -> myMux Fun4/2(u2)
  Demux/3 -> myMux Fun4/3(u3)
  Demux/4 -> myMux Fun4/4(u4)
  Demux/5 -> myMux Fun4/5(u5)
  Demux/6 -> myMux Fun4/6(u6)
  Demux1/1 -> myMux Fun4/7(u7)
  Demux1/2 -> myMux Fun4/8(u8)
  Demux1/3 -> myMux Fun4/9(u9)
  Constant/1 -> Embedded MATLAB Function/1(u)  "Baro"
  Constant1/1 -> Embedded MATLAB Function1/1(u)  "Pitot"
  Constant2/1 -> Embedded MATLAB Function2/1(u)  "Power"
  Constant3/1 -> Embedded MATLAB Function3/1(u)  "Thermistor"
  myMux Fun/1(y) -> Update State AP ADC Data [updateSensorMcuState.c]1/1
  Data Type Conversion/1 -> myMux Fun4/10(u10), myMux Fun/1(u1)
  Data Type Conversion1/1 -> myMux Fun4/11(u11), myMux Fun/2(u2)
  Data Type Conversion2/1 -> myMux Fun4/12(u12), myMux Fun/3(u3)
  Data Type Conversion3/1 -> myMux Fun4/13(u13), myMux Fun/4(u4)
  Embedded MATLAB Function1/1(y) -> Data Type Conversion1/1
  Embedded MATLAB Function2/1(y) -> Data Type Conversion2/1
  Read the Cube Data [adisCube16405.c]1/1 -> Demux2/1
  Demux2/3 -> Terminator/1
  Demux2/2 -> Demux1/1
  From4/1 -> Switch2/2
  Is the GPS Novatel or Ublox? [gpsPort.c]1/1 -> Logical Operator/1
  if GPS is Novatel/1(GPS Main) -> Switch2/1
  Logical Operator/1 -> [isUblox]
  From1/1 -> if GPS is Novatel/Enable
  [isUblox] -> if GPS is Ublox/Enable
  if GPS is Ublox/1(GPS Main) -> GPS/1
  Get RawGpsInt/1 -> Data Type Conversion4/1
  Get RawGpsInt/2 -> Data Type Conversion5/1
  Get RawGpsInt/3 -> Data Type Conversion6/1
  Get RawGpsInt/4 -> Data Type Conversion8/1
  Get RawGpsInt/5 -> Data Type Conversion9/1
  Data Type Conversion4/1 -> Bus Creator3/1
  Data Type Conversion5/1 -> Bus Creator3/2
  Data Type Conversion6/1 -> Bus Creator3/3
  Data Type Conversion8/1 -> Bus Creator3/4
  Data Type Conversion9/1 -> Bus Creator3/5
  Bus Creator3/1 -> ?
  Get Raw IMU/1 -> Bus Creator/1
  Get Raw IMU/2 -> Bus Creator/2
  Get Raw IMU/3 -> Bus Creator/3
  Get Raw IMU/4 -> Bus Creator1/1
  Get Raw IMU/5 -> Bus Creator1/2
  Get Raw IMU/6 -> Bus Creator1/3
  Get Raw IMU/7 -> Bus Creator2/1
  Get Raw IMU/8 -> Bus Creator2/2
  Get Raw IMU/9 -> Bus Creator2/3
  Get mlAirData1/1 -> Data Type Conversion/1
  Get mlAirData2/1 -> Data Type Conversion3/1

== system SLUGS2/Sensor_Data_Adapter/Sensor Suite/If no HIL then update Air Data ==
  AirData : Inport
  Enable : EnablePort
  Demux : Demux  Outputs=[1 2]
  Terminator : Terminator
  Update the Air Calibrated Data [updateSensorMcuState.c]1 : MCHP_Blockset/User Functions/C Function Call  ParseFilesChkbx=off  ListFunctions1=Custom Function  Function1=extern void updateAirData(real32_T* u1);  AddHeaderDeclaration=on  Function1Type=when block is updated (default)  FctReturnBlockOut=off  DataCollected=0  ORDERING=None  SampleTime=.01  MCHP_MASTERLINK=|  PinDigitalInput=[]  PinDigitalOutput=[]  PinAnalogInput=[]
      | SLUGS2/Microchip Master
      | AUAV V3 Board
      | Busy Flag on D2 (RA6)
  Out1 : Outport
  wires:
  AirData/1 -> Demux/1, Update the Air Calibrated Data [updateSensorMcuState.c]1/1
  Demux/1 -> Out1/1
  Demux/2 -> Terminator/1
